simulink model "PipeHeatX"  (R2015a)
settings: Solver=FixedStepDiscrete  StartTime=0.0  StopTime=tsim  FixedStep=dt  RelTol=1e-3
values from neighbouring files (symbols this model uses):
  Cp = 6.92*ones(length(r),1)'    [run_PipeHeatX.m]
  Cpin = 32.3*778.169    (= 25134.8587)    [run_PipeHeatX.m]
  Din = r(1)*2    [run_PipeHeatX.m]
  Dout = r(end)*2    [run_PipeHeatX.m]
  k = 0.0328*ones(length(r),1)'    [run_PipeHeatX.m]
  kin = 0.0001076*778.169    (= 0.0837309844)    [run_PipeHeatX.m]
  muin = 1.86*10^-5    (= 1.86e-05)    [run_PipeHeatX.m]
  r = linspace(1/12,1.5/12,20)    [run_PipeHeatX.m]
  rho = 5.238864896*ones(length(r),1)'    [run_PipeHeatX.m]
  rhoin = 1.94    [run_PipeHeatX.m]
  rhoout = 0.00237    [run_PipeHeatX.m]
  Tin = 654    [run_PipeHeatX.m]
  To = 550*ones(length(r),1)'    [run_PipeHeatX.m]
  Tout = 460    [run_PipeHeatX.m]
  velin = 1    [run_PipeHeatX.m]
  velout = 50    [run_PipeHeatX.m]
libraries: lib_Convection_NonDimParms x3, lib_AirProps_HeatCapacity x2, lib_AirProps_ThermCond x2, lib_AirProps_Viscosity x2, lib_Conduction_HeatX1DVarPropsAndGenBCs x1, lib_Convection_Gnielinski x1, lib_Convection_CylCrossFlowZukauskas x1
settings Model: Creator=jlkratz  LastModifiedBy=jlkratz

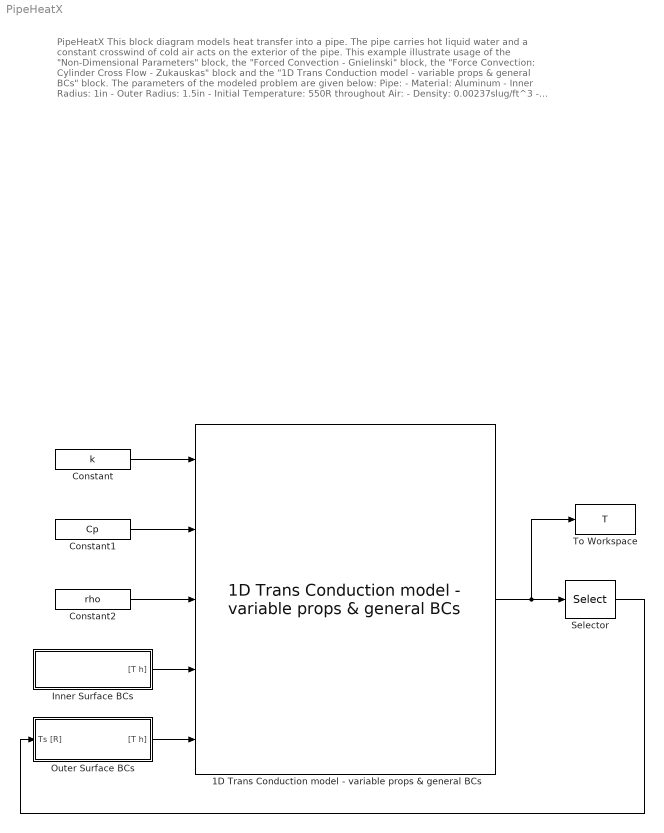
== system PipeHeatX ==
  note: PipeHeatX
      |
      | This block diagram models heat transfer into a pipe. The pipe carries hot liquid water and a constant
      | crosswind of cold air acts on the exterior of the pipe. This example illustrate usage of the
      | "Non-Dimensional Parameters" block, the "Forced Convection - Gnielinski" block, the
      | "Force Convection: Cylinder Cross Flow - Zukauskas" block and the "1D Trans Conduction model -
      | variable props & general BCs" block. The parameters of the modeled problem are given below:
      | Pipe:
      | - Material: Aluminum
      | - Inner Radius: 1in
      | - Outer Radius: 1.5in
      | - Initial Temperature: 550R throughout
      | Air:
      | - Density: 0.00237slug/ft^3
      | - Temperature: 460R
      | - Velocity: 50ft/sec
      | Water:
      | Density: 1.94slug/ft^3
      | Temperature: 654R
      | Heat Capacity: 32.3Btu/(slug-R)
      | Thermal Conductivity: 0.0001076Btu/(sec-ft-R)
      | Viscosity: 1.86*10^-5slug/(ft-sec)
      | Velocity: 1ft/sec
  1D Trans Conduction model - variable props & general BCs : lib_Conduction_HeatX1DVarPropsAndGenBCs/1D Trans Conduction model - variable props & general BCs  x_M=r  T0_M=To  dt_M=dt  a_M=on  convin_M=on  radin_M=off  condin_M=off  convout_M=on  radout_M=off  condout_M=off  BN_M=double(gcb)
  Constant : Constant  Value=k
  Constant1 : Constant  Value=Cp
  Constant2 : Constant  Value=rho
  Inner Surface BCs : Subsystem
  Outer Surface BCs : Subsystem
  Selector : Selector  InputPortWidth=length(r)  Indices=length(r)
  To Workspace : ToWorkspace  VariableName=T  SaveFormat=Timeseries  SampleTime=-1
  wires:
  Constant/1 -> 1D Trans Conduction model - variable props & general BCs/1
  Constant1/1 -> 1D Trans Conduction model - variable props & general BCs/2
  Constant2/1 -> 1D Trans Conduction model - variable props & general BCs/3
  Inner Surface BCs/1("[T h]") -> 1D Trans Conduction model - variable props & general BCs/4
  1D Trans Conduction model - variable props & general BCs/1 -> To Workspace/1, Selector/1
  Selector/1 -> Outer Surface BCs/1(Ts [R])
  Outer Surface BCs/1("[T h]") -> 1D Trans Conduction model - variable props & general BCs/5

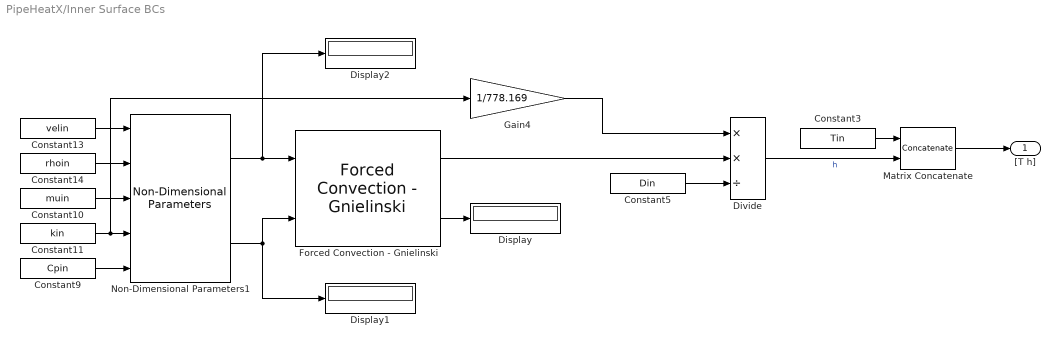
== system PipeHeatX/Inner Surface BCs ==
  Constant10 : Constant  Value=muin
  Constant11 : Constant  Value=kin
  Constant13 : Constant  Value=velin
  Constant14 : Constant  Value=rhoin
  Constant3 : Constant  Value=Tin
  Constant5 : Constant  Value=Din
  Constant9 : Constant  Value=Cpin
  Display : Display
  Display1 : Display
  Display2 : Display
  Divide : Product  Inputs=**/
  Forced Convection - Gnielinski : lib_Convection_Gnielinski/Forced Convection - Gnielinski  SmoothOrRough_M=Smooth  eoD_M=[0.02 0.01]
  Gain4 : Gain  Gain=1/778.169
  Matrix Concatenate : Concatenate  ConcatenateDimension=2
  Non-Dimensional Parameters1 : lib_Convection_NonDimParms/Non-Dimensional Parameters  M_M=off  Re_M=on  Pr_M=on  Gr_M=off  Ra_M=off  Bi_M=off  Fo_M=off  Nu_M=off  St_M=off  Ec_M=off  jH_M=off  Pe_M=off  perfGas_M=off  R_M=1716  mdot_A_or_rhov_M=off  A_M=1  L_M=Din  g_M=32.174  t_M=1
  "[T h]" : Outport
  wires:
  Forced Convection - Gnielinski/2 -> Display/1
  Constant3/1 -> Matrix Concatenate/1
  Constant10/1 -> Non-Dimensional Parameters1/3
  Constant9/1 -> Non-Dimensional Parameters1/5
  Constant11/1 -> Gain4/1, Non-Dimensional Parameters1/4
  Non-Dimensional Parameters1/2 -> Forced Convection - Gnielinski/2, Display1/1
  Constant5/1 -> Divide/3
  Constant14/1 -> Non-Dimensional Parameters1/2
  Constant13/1 -> Non-Dimensional Parameters1/1
  Matrix Concatenate/1 -> "[T h]"/1
  Forced Convection - Gnielinski/1 -> Divide/2
  Non-Dimensional Parameters1/1 -> Display2/1, Forced Convection - Gnielinski/1
  Divide/1 -> Matrix Concatenate/2  "h"
  Gain4/1 -> Divide/1

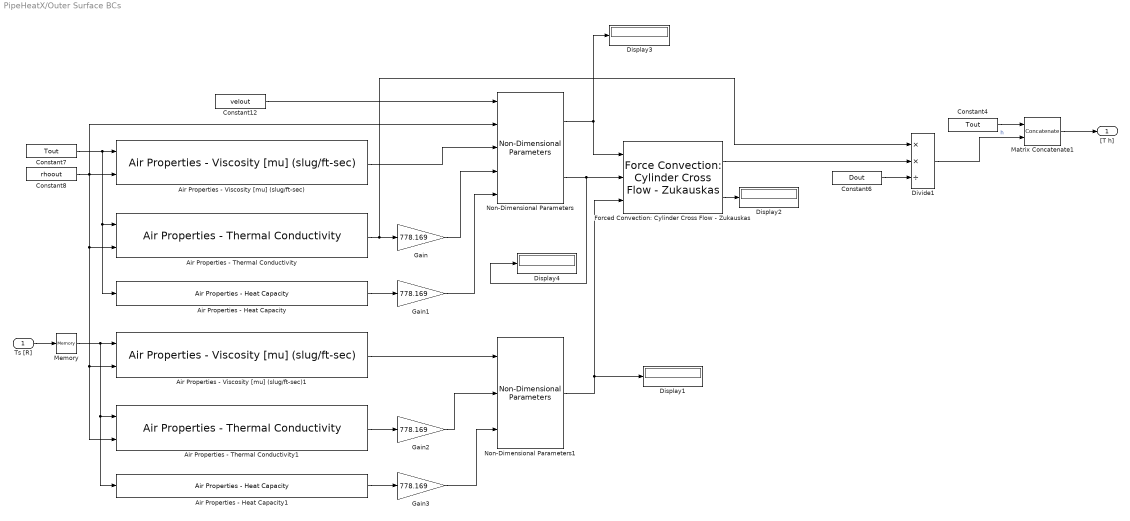
== system PipeHeatX/Outer Surface BCs ==
  Ts [R] : Inport
  Air Properties - Heat Capacity : lib_AirProps_HeatCapacity/Air Properties - Heat Capacity  BN_M=double(gcb)
  Air Properties - Heat Capacity1 : lib_AirProps_HeatCapacity/Air Properties - Heat Capacity  BN_M=double(gcb)
  Air Properties - Thermal Conductivity : lib_AirProps_ThermCond/Air Properties - Thermal Conductivity  BN_M=double(gcb)
  Air Properties - Thermal Conductivity1 : lib_AirProps_ThermCond/Air Properties - Thermal Conductivity  BN_M=double(gcb)
  Air Properties - Viscosity [mu] (slug/ft-sec) : lib_AirProps_Viscosity/Air Properties - Viscosity [mu] (slug//ft-sec)  BN_M=double(gcb)
  Air Properties - Viscosity [mu] (slug/ft-sec)1 : lib_AirProps_Viscosity/Air Properties - Viscosity [mu] (slug//ft-sec)  BN_M=double(gcb)
  Constant12 : Constant  Value=velout
  Constant4 : Constant  Value=Tout
  Constant6 : Constant  Value=Dout
  Constant7 : Constant  Value=Tout
  Constant8 : Constant  Value=rhoout
  Display{1..4} (4 alike) : Display
  Divide1 : Product  Inputs=**/
  Forced Convection: Cylinder Cross Flow - Zukauskas : lib_Convection_CylCrossFlowZukauskas/Force Convection: Cylinder Cross Flow  - Zukauskas
  Gain{,1..3} (4 alike) : Gain  Gain=778.169
  Matrix Concatenate1 : Concatenate  ConcatenateDimension=2
  Memory : Memory  X0=To(length(r))
  Non-Dimensional Parameters : lib_Convection_NonDimParms/Non-Dimensional Parameters  M_M=off  Re_M=on  Pr_M=on  Gr_M=off  Ra_M=off  Bi_M=off  Fo_M=off  Nu_M=off  St_M=off  Ec_M=off  jH_M=off  Pe_M=off  perfGas_M=on  R_M=1716  mdot_A_or_rhov_M=off  A_M=1  L_M=Dout  g_M=32.174  t_M=1
  Non-Dimensional Parameters1 : lib_Convection_NonDimParms/Non-Dimensional Parameters  M_M=off  Re_M=off  Pr_M=on  Gr_M=off  Ra_M=off  Bi_M=off  Fo_M=off  Nu_M=off  St_M=off  Ec_M=off  jH_M=off  Pe_M=off  perfGas_M=on  R_M=1716  mdot_A_or_rhov_M=off  A_M=1  L_M=1  g_M=32.174  t_M=1
  "[T h]" : Outport
  wires:
  Constant12/1 -> Non-Dimensional Parameters/1
  Matrix Concatenate1/1 -> "[T h]"/1
  Air Properties - Viscosity [mu] (slug/ft-sec)1/1 -> Non-Dimensional Parameters1/1
  Memory/1 -> Air Properties - Heat Capacity1/1, Air Properties - Thermal Conductivity1/1, Air Properties - Viscosity [mu] (slug/ft-sec)1/1
  Forced Convection: Cylinder Cross Flow - Zukauskas/2 -> Display2/1
  Constant6/1 -> Divide1/3
  Forced Convection: Cylinder Cross Flow - Zukauskas/1 -> Divide1/2
  Constant7/1 -> Air Properties - Heat Capacity/1, Air Properties - Thermal Conductivity/1, Air Properties - Viscosity [mu] (slug/ft-sec)/1
  Constant8/1 -> Non-Dimensional Parameters/2, Air Properties - Thermal Conductivity1/2, Air Properties - Viscosity [mu] (slug/ft-sec)1/2, Air Properties - Thermal Conductivity/2, Air Properties - Viscosity [mu] (slug/ft-sec)/2
  Air Properties - Heat Capacity/1 -> Gain1/1
  Non-Dimensional Parameters/1 -> Forced Convection: Cylinder Cross Flow - Zukauskas/1, Display3/1
  Air Properties - Viscosity [mu] (slug/ft-sec)/1 -> Non-Dimensional Parameters/3
  Divide1/1 -> Matrix Concatenate1/2  "h"
  Constant4/1 -> Matrix Concatenate1/1
  Non-Dimensional Parameters/2 -> Display4/1, Forced Convection: Cylinder Cross Flow - Zukauskas/2
  Air Properties - Heat Capacity1/1 -> Gain3/1
  Air Properties - Thermal Conductivity1/1 -> Gain2/1
  Ts [R]/1 -> Memory/1
  Non-Dimensional Parameters1/1 -> Display1/1, Forced Convection: Cylinder Cross Flow - Zukauskas/3
  Gain/1 -> Non-Dimensional Parameters/4
  Gain1/1 -> Non-Dimensional Parameters/5
  Gain2/1 -> Non-Dimensional Parameters1/2
  Gain3/1 -> Non-Dimensional Parameters1/3
  Air Properties - Thermal Conductivity/1 -> Divide1/1, Gain/1
